simulink model "Drive_Machine"  (R2025a)
settings: Solver=ode23s  StartTime=0.0  StopTime=0.5  MaxStep=1e-5  RelTol=1e-3  AbsTol=1e-3  EnableMultiTasking=on
values from neighbouring files (symbols this model uses):
  f_r = 20    [ISCAD_Analytical.m]
  mparams = load_json_parameters('../ISCAD_parameters.json')    [ISCAD_Analytical.m]    (also in ISCAD_Coupled_Model.m = struct(); PowerElectronics_Analytical.m = load_json_parameters('../TEST_parameters.json'); load_json_parameters.m = struct(); simulik_parameter_setter_inverter.m = load_json_parameters('../TEST_parameters.json'))
  Td = 2e-6    (= 2e-06)    [PowerElectronics_Analytical.m]    (also in simulik_parameter_setter_inverter.m)
  Vs_rms = 0.03    [ISCAD_Analytical.m]
undefined symbols (not defined in the file or in its folder): inv, mach, mi_idx, omega_idx, T, T_sample
libraries: nesl_utility x14, fl_lib x11, ee_lib x5, eePwmGeneratorTwoLevel x1, spsRMSLib x1, simulink x1, spsThreePhaseSineGeneratorLib x1
Description:
  | Three-Phase Voltage-Sourced Converter (SPWM)
  | 
  | This example shows how to model a three-phase voltage-sourced
  | converter that uses Sinusoidal Pulse-Width Modulation (SPWM).
  | This modulation scheme compares a reference sine wave with a
  | higher-frequency repeating triangle wave in order to generate the
  | pulses. The model can be used to support selection of suitable
  | values for L, C and the pulse modulation scheme parameters.
settings Model: Creator=The MathWorks, Inc.  LastModifiedBy=aj22365
settings SolverCC: AutoScaleAbsTol=off  ZeroCrossAlgorithm=Adaptive  AlgebraicLoopSolver=TrustRegion
settings DataIOCC: LimitDataPoints=on  SaveFormat=Array  ReturnWorkspaceOutputs=off
settings OptimizationCC: LifeSpan=inf
settings DebuggingCC: UnderspecifiedInitializationDetection=Classic  MergeDetectMultiDrivingBlocksExec=none  IgnoredZcDiagnostic=none  SolverPrmCheckMsg=warning  UnconnectedInputMsg=warning  UnconnectedOutputMsg=warning  UnconnectedLineMsg=warning  PregeneratedLibrarySubsystemCodeDiagnostic=none  SFUnexpectedBacktrackingDiag=warning  SFNoUnconditionalDefaultTransitionDiag=warning  SFExecutionAtInitializationDiag=none  ArithmeticOperatorsInVariantConditions=warning
settings HardwareCC: ProdBitPerPointer=32.0  ProdBitPerSizeT=32.0  ProdBitPerPtrDiffT=32.0  ProdLargestAtomicFloat=None  ProdIntDivRoundTo=Undefined  ProdEndianess=Unspecified  ProdWordSize=32.0  ProdHWDeviceType=32-bit Generic
settings ModelReferenceCC: EnableRefExpFcnMdlSchedulingChecks=on  PropagateSignalLabelsOutOfModel=off
settings SFSimCC: SimUseLocalCustomCode=off  CustomCodeUndefinedFunction=UseInterfaceOnly
settings RTWCC: RTWUseLocalCustomCode=off  GPUComputeCapability=3.5
settings CodeAppCC: StateflowObjectComments=on
settings GRTTargetCC: TargetLangStandard=C89/C90 (ANSI)
settings ConfigComp: CovMetricSettings=dw  CovSaveCumulativeToWorkspaceVar=on  CovSaveSingleToWorkspaceVar=on  CovExternalEMLEnable=off  CovSFcnEnable=off
settings SimscapeCC: SimscapeNormalizeSystem=off

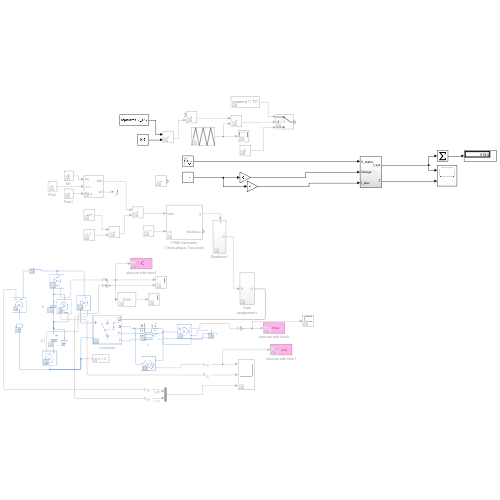
[thumbnail: Simulink's stored preview of the top-level diagram]
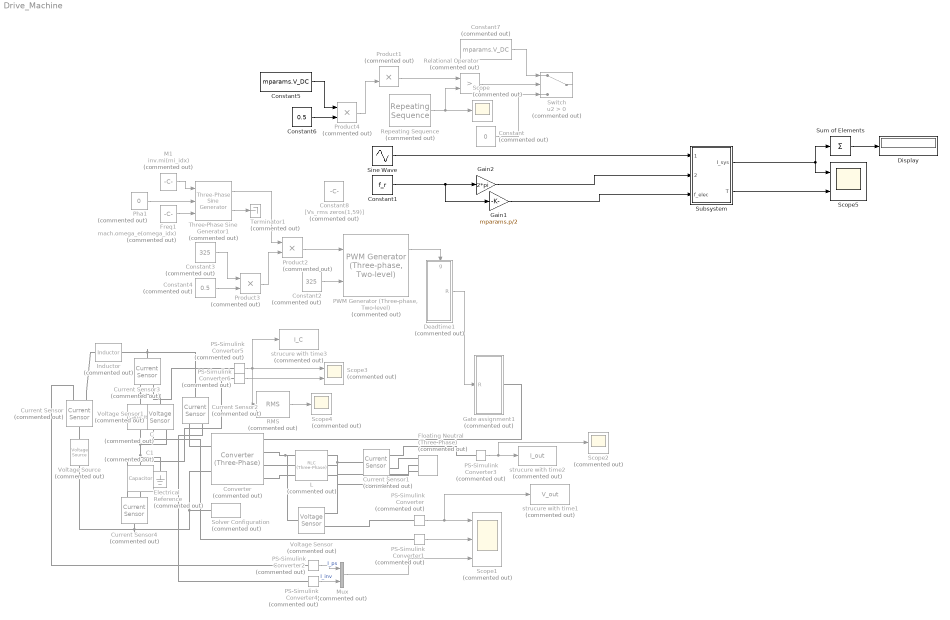
== system Drive_Machine ==
  C : fl_lib/Electrical/Electrical Elements/Capacitor  Commented=on  c=5000 uF  r=0 Ohm  g=0 1/Ohm  i_specify=off  i_priority=High  i=0 A  i_nominal_specify=off  i_nominal_value=1  i_nominal_unit=A  v_specify=on  v_priority=None  v=46 V  v_nominal_specify=off  v_nominal_value=1  v_nominal_unit=V  vc_specify=off  vc_priority=High  vc=0 V  vc_nominal_specify=off  vc_nominal_value=1  vc_nominal_unit=V
  C1 : fl_lib/Electrical/Electrical Elements/Capacitor  Commented=on  c=5000 uF  r=0 Ohm  g=0 1/Ohm  i_specify=off  i_priority=High  i=0 A  i_nominal_specify=off  i_nominal_value=1  i_nominal_unit=A  v_specify=on  v_priority=None  v=46 V  v_nominal_specify=off  v_nominal_value=1  v_nominal_unit=V  vc_specify=off  vc_priority=High  vc=0 V  vc_nominal_specify=off  vc_nominal_value=1  vc_nominal_unit=V
  Constant : Constant  Commented=on  Value=0
  Constant1 : Constant  Value=f_r
  Constant2 : Constant  Commented=on  Value=325
  Constant3 : Constant  Commented=on  Value=325
  Constant4 : Constant  Commented=on  Value=0.5
  Constant5 : Constant  Value=mparams.V_DC
  Constant6 : Constant  Value=0.5
  Constant7 : Constant  Commented=on  Value=mparams.V_DC
  Constant8 : Constant  Commented=on  Value=[Vs_rms zeros(1,59)]
  Converter : ee_lib/Semiconductors & Converters/Converters/Converter (Three-Phase)  Commented=on  port_option=ee.enum.threePhasePort.expanded  fidelity_option=ee.enum.converters.fidelity.detailed  device_type=ee.enum.converters.switchingdevice.igbt  showThermalPort=false  K=0  Vth=0.5 V  Vgt=0.5 V  Vgt_off=0.1 V  Ih=1 A  Vf=0.6 V  Ron=0.002 Ohm  Rds=0.002 Ohm  Goff=1e-6 S  Eon_scalar=22.86e-3 J  Eoff_scalar=17.14e-3 J  Eoff_natural_commutation=10e-3 J  Voff=300 V  Iout_scalar=600 A  onCurrentMeasDelay=0 s  useCurrentFromPreviousCycle=false  useVoltageFromPreviousCycle=false  diode_param=2  diode_Vf=0.8 V  diode_Ron=0.001 Ohm  diode_Goff=1e-5 S  diode_C=5e-8 F  diode_iRM=-235 A  diode_iF=300 A  diode_idot=-50 A/us  diode_trr_param=1  diode_trr_factor=3  diode_trr=15 us  diode_Qrr=1.5e+3 s*uA  diode_rec_loss_model=ee.enum.diode.reverseRecoveryModel.fixed  diode_ErecVal=0 J  diode_scaleWithIandV=false  diode_ErecMat=zeros(2, 3) J  diode_TjrecVec=[298.15, 398.15] K  diode_IfrecVec=[.1, 1, 10] A  diode_IrecVal=10 A  diode_VrecVal=10 V  diode_tFilter=1 / 1000 / 100 s  thermal_network_parameterization=ee.enum.thermalNetworkTopology.external  Rth=[.08, .5] K/W  Rth_Cauer=[.08, .1, .5] K/W  Rth_Foster=[.08, .14, .22, .16] K/W  thermal_mass_parameterization=ee.enum.thermalNetwork.timeconstant  thermal_mass=[.01, .5] J/K  thermal_mass_Cauer=[.01, .1, .5] J/K  thermal_mass_Foster=[.001, .005, .05, .5] J/K  thermal_time_constant=[.001, .2] s  thermal_time_constant_Cauer=[.001, .1, .2] s  thermal_time_constant_Foster=[7e-05, .0007, .01, .08] s  thermal_mass_initial_temperatures=[25, 25] degC  thermal_mass_initial_temperatures_Cauer=[25, 25, 25] degC  junction_thermal_mass=0.01 J/K  Tvec_initial_Foster=[25, 25, 25, 25] degC  snubber_type=0  Cs=1e-7 F  Rs=0.1 Ohm  Vce_loss=[0, 150, 300] V
      settings: InternalSimscapePortConfiguration="{\"Bottom\":[],\"Left\":[{\"id\":\"G\",\"label\":\"G\",\"type\":\"foundation.electrical.twelve_phase\"},{\"id\":\"a\",\"label\":\"a\",\"type\":\"foundation.electrical.electrical\"},{\"id\":\"b\",\"label\":\"b\",\"type\":\"foundation.electrical.electrical\"},{\"id\":\"c\",\"label\":\"c\",\"type\":\"foundation.electrical.electrical\"}],\"Right\":[{\"id\":\"p\",\"label\":\"+\",\"type\":\"foundation.electrical.electrical\"},{\"id\":\"n\",\"label\":\"-\",\"type\":\"foundation.electrical.electrical\"}],\"Top\":[]}"
  Current Sensor{,1..4} (5 alike) : fl_lib/Electrical/Electrical Sensors/Current Sensor  Commented=on
  Deadtime1 : Subsystem  Commented=on
      settings: PortSchema="{\"entries\":[{\"content\":{\"sides\":[{\"content\":{\"connectorIds\":[\"Out1\"]},\"type\":\"ConnectorPlacement.EquallySpacedRectSide\",\"uuid\":\"80ef36b9-f465-4fcc-93a9-9d6eab044ae8\"},{\"content\":{\"side\":\"RIGHT\"},\"type\":\"ConnectorPlacement.EquallySpacedRectSide\",\"uuid\":\"10827d79-0026-467d-af8f-e653363972a6\"},{\"content\":{\"connectorIds\":[\"In1\"],\"side\":\"TOP\"},\"type\":\"ConnectorPlacement.EquallySpacedRectSide\",\"uuid\":\"d9163dac-283f-4784-a2ff-48ce53974a1a\"}]},\"type\":\"ConnectorPlacement.EquallySpacedConnector\",\"uuid\":\"7e643ad6-bdf3-49e0-97a6-0ece4f3a3f1f\"}],\"packageUris\":[\"http://schema.mathworks.com/mf0/Connector/R2020b\"],\"version\":\"1.0\"}"
  Display : Display
  Electrical Reference : fl_lib/Electrical/Electrical Elements/Electrical Reference  Commented=on
  Floating Neutral (Three-Phase) : ee_lib/Connectors & References/Floating Neutral (Three-Phase)  Commented=on  G_parasitic=1e-12 1/Ohm
      settings: InternalSimscapePortConfiguration="{\"Bottom\":[],\"Left\":[{\"id\":\"a\",\"label\":\"a\",\"type\":\"foundation.electrical.electrical\"},{\"id\":\"b\",\"label\":\"b\",\"type\":\"foundation.electrical.electrical\"},{\"id\":\"c\",\"label\":\"c\",\"type\":\"foundation.electrical.electrical\"}],\"Right\":[],\"Top\":[]}"
  Freq1 : Constant  Commented=on  Value=mach.omega_e(omega_idx)
  Gain1 : Gain  Gain=mparams.p/2
  Gain2 : Gain  Gain=2*pi
  Gate assignment1 : Subsystem  Commented=on
  Inductor : fl_lib/Electrical/Electrical Elements/Inductor  Commented=on  l=0.000008 H  r=0.05 Ohm  g=1e-9 1/Ohm  i_specify=on  i_priority=None  i=2 A  i_nominal_specify=off  i_nominal_value=1  i_nominal_unit=A  v_specify=off  v_priority=None  v=0 V  v_nominal_specify=off  v_nominal_value=1  v_nominal_unit=V  i_L_specify=on  i_L_priority=High  i_L=2 A  i_L_nominal_specify=off  i_L_nominal_value=1  i_L_nominal_unit=A
  L : ee_lib/Passive/RLC Assemblies/RLC (Three-Phase)  Commented=on  port_option=ee.enum.threePhasePort.expanded  component_structure=4  R=.054 Ohm  L=.00285 H  C=1e-6 F  R_parasitic=1e-6 Ohm  G_parasitic=1e-6 1/Ohm  IL_specify=on  IL_priority=High  IL=[ -14 7 7 ] A  IL_nominal_specify=off  IL_nominal_value=1  IL_nominal_unit=A  VC_specify=on  VC_priority=High  VC=[ 0 0 0 ] V  VC_nominal_specify=off  VC_nominal_value=1  VC_nominal_unit=V
      settings: InternalSimscapePortConfiguration="{\"Bottom\":[],\"Left\":[{\"id\":\"a1\",\"label\":\"a1\",\"type\":\"foundation.electrical.electrical\"},{\"id\":\"b1\",\"label\":\"b1\",\"type\":\"foundation.electrical.electrical\"},{\"id\":\"c1\",\"label\":\"c1\",\"type\":\"foundation.electrical.electrical\"}],\"Right\":[{\"id\":\"a2\",\"label\":\"a2\",\"type\":\"foundation.electrical.electrical\"},{\"id\":\"b2\",\"label\":\"b2\",\"type\":\"foundation.electrical.electrical\"},{\"id\":\"c2\",\"label\":\"c2\",\"type\":\"foundation.electrical.electrical\"}],\"Top\":[]}"
  M1 : Constant  Commented=on  Value=inv.mi(mi_idx)
  Mux : Mux  Commented=on  Inputs=2
  PS-Simulink Converter{,1..6} (7 alike) : nesl_utility/PS-Simulink Converter  Commented=on  PhysicalDomain=network_engine_domain  SubClassName=ps_output  LeftPortType=input  RightPortType=output  PseudoPeriodic=off  Frequencies=[]  VectorFormat=inherit  Unit=inherit  AffineConversion=off
  "PWM Generator (Three-phase, Two-level)" : eePwmGeneratorTwoLevel/PWM Generator (Three-phase, Two-level)  Commented=on  PWMMode=Continuous PWM (CPWM)  CPWMMode=SPWM: sinusoidal PWM  DPWMMode=30 DPWM: 30 degree discontinuous PWM  fsw=f_s  Ts=T
      settings: SamplingMode=Asymmetric
      settings: LibrarySourceBlock=|
      | ee_sl_lib/Pulse Width
      | Modulation/PWM Generator
      | (Three-phase, Two-level)
  Pha1 : Constant  Commented=on  Value=0
  Product{1..4} (4 alike) : Product  Commented=on
  RMS : spsRMSLib/RMS  Commented=on  TrueRMS=on  Freq=25  RMSInit=0  Ts=inv.T_s
  Relational Operator : RelationalOperator  Commented=on  Operator=>  OutDataTypeStr=boolean  RndMeth=Simplest  InputSameDT=off
  Repeating Sequence : simulink/Sources/Repeating Sequence  Commented=on  rep_seq_t=[0, 1/mparams.f_sw/2, 1/mparams.f_sw]  rep_seq_y=[-1, 1, -1]
  Scope : Scope  Commented=on
      settings: ActiveDisplayYMinimum=-1.25  ActiveDisplayYMaximum=1.25  DataLoggingVariableName=ScopeData3
  Scope1 : Scope  Commented=on  NumInputPorts=3
      settings: ActiveDisplayYMinimum=-286.10507  ActiveDisplayYMaximum=270.03945
  Scope2 : Scope  Commented=on
      settings: ActiveDisplayYMinimum=-372.34194  ActiveDisplayYMaximum=490.06934  DataLoggingVariableName=ScopeData2
  Scope3 : Scope  Commented=on  NumInputPorts=2
      settings: ActiveDisplayYMinimum=-411.29295  ActiveDisplayYMaximum=631.29859
  Scope4 : Scope  Commented=on
      settings: ActiveDisplayYMinimum=-372.34194  ActiveDisplayYMaximum=490.06934
  Scope5 : Scope  NumInputPorts=2
      settings: ActiveDisplayYMinimum=-2.2013460421337228  ActiveDisplayYMaximum=19.812114379203507
  Sine Wave : Sin  Amplitude=Vs_rms*sqrt(2)/mparams.V_DC  Bias=2*Vs_rms*sqrt(2)/mparams.V_DC  Frequency=f_r*mparams.p/2  Phase=[(0:(mparams.Qs-1))*2*pi/60]'  SampleTime=0  VectorParams1D=off
  Solver Configuration : nesl_utility/Solver Configuration  Commented=on  PhysicalDomain=network_engine_domain  SubClassName=solver  LeftPortType=input  RightPortType=generic  Tones=[]  Harmonics=[]  SimulateNoise=off  Profile=off  UseLocalSampling=off  EnableSwitchedLinearOptims=on  FrequencyDomain=off  UseCCode=off  RelTol=0.001  AbsTol=1e-06  MinStep=1e-09  ToWorkspace=off  RevertToSquareIcSolve=off  NumHomotopyIterations=100  PhasorMode=off  PhasorModeNumHarmonics=1  ConsistencySolver=NEWTON_FTOL  IndexReductionMethod=DerivativeReplacement  DoDC=off  ResidualTolerance=1e-09  ConsistencyTolSource=GLOBAL  ConsistencyAbsTol=0.001  ConsistencyRelTol=0.001  ConsistencyTolFactor=0.001  UseLocalSolver=off  LocalSolverChoice=NE_BACKWARD_EULER_ADVANCER  ResolveIndetEquations=on  FunctionEvalNumThread=1  LocalSolverSampleTime=1e-5  DoFixedCost=off  MaxNonlinIter=5  MaxModeIter=2  ComputeImpulses=off  ImpulseIterations=2  LinearAlgebra=Sparse  LinearAlgebraNumThread=0  EquationFormulation=NE_TIME_EF  DelaysMemoryBudget=1024  AutomaticFiltering=on  FilteringTimeConstant=0.001  PartitionStorageMethod=AS_NEEDED  PartitionMemoryBudget=1024  PartitionMethod=FAST  MultibodyUseLocalSolver=off  MultibodyLocalSolverChoice=ODE1  MultibodyLocalSolverSampleTime=0.001
  Subsystem : Subsystem
  Sum of Elements : Sum  Inputs=+
  Switch : Switch  Commented=on  Criteria=u2 > Threshold  SaturateOnIntegerOverflow=off  InputSameDT=off
  Terminator1 : Terminator  Commented=on
  Three-Phase Sine Generator1 : spsThreePhaseSineGeneratorLib/Three-Phase Sine Generator  Commented=on  Ts=T
      settings: LibrarySourceBlock=|
      | sps_lib/Sources/Signal Generator Sources/Three-Phase
      | Sine Generator
  Voltage Sensor : fl_lib/Electrical/Electrical Sensors/Voltage Sensor  Commented=on
  Voltage Sensor1 : fl_lib/Electrical/Electrical Sensors/Voltage Sensor  Commented=on
  Voltage Source : ee_lib/Sources/Voltage Source  Commented=on  dc_voltage=325 V  ac_voltage=0 V  ac_shift=0 rad  ac_frequency=0 Hz  noise_mode=ee.enum.sources.noise.Disabled  PSD=0 V^2/Hz  sample_time=1e-3 s  repeatability=ee.enum.sources.repeatability.NotRepeatable  user_seed=0  auto_seed=3890346746  i_specify=off  i_priority=None  i=0 A  i_nominal_specify=off  i_nominal_value=1  i_nominal_unit=A  v_specify=off  v_priority=None  v=0 V  v_nominal_specify=off  v_nominal_value=1  v_nominal_unit=V
  strucure with time1 : ToWorkspace  Commented=on  VariableName=V_out  SaveFormat=Structure With Time  SampleTime=T_sample
  strucure with time2 : ToWorkspace  Commented=on  VariableName=I_out  SaveFormat=Structure With Time  SampleTime=T_sample
  strucure with time3 : ToWorkspace  Commented=on  VariableName=I_C  SaveFormat=Structure With Time  SampleTime=T_sample
  wires:
  Pha1/1 -> Three-Phase Sine Generator1/2
  Constant2/1 -> "PWM Generator (Three-phase, Two-level)"/2
  Product3/1 -> Product2/2
  Freq1/1 -> Three-Phase Sine Generator1/3
  Constant4/1 -> Product3/2
  Three-Phase Sine Generator1/2 -> Terminator1/1
  M1/1 -> Three-Phase Sine Generator1/1
  Product2/1 -> "PWM Generator (Three-phase, Two-level)"/1
  Constant3/1 -> Product3/1
  Three-Phase Sine Generator1/1 -> Product2/1
  PS-Simulink Converter/1 -> strucure with time1/1, Scope1/1
  Deadtime1/1(R) -> Gate assignment1/1(R)
  "PWM Generator (Three-phase, Two-level)"/1 -> Deadtime1/1(g)
  PS-Simulink Converter1/1 -> Scope1/2
  PS-Simulink Converter3/1 -> Scope2/1, strucure with time2/1
  PS-Simulink Converter4/1 -> Mux/2  "I_inv"
  PS-Simulink Converter2/1 -> Mux/1  "I_ps"
  Mux/1 -> Scope1/3
  PS-Simulink Converter6/1 -> Scope3/2
  PS-Simulink Converter5/1 -> strucure with time3/1, RMS/1, Scope3/1
  RMS/1 -> Scope4/1
  Constant1/1 -> Gain1/1, Gain2/1
  Sum of Elements/1 -> Display/1
  Subsystem/1(I_sys) -> Sum of Elements/1, Scope5/1
  Gain2/1 -> Subsystem/2(Omega)
  Gain1/1 -> Subsystem/3(f_elec)
  Subsystem/2(T) -> Scope5/2
  Constant6/1 -> Product4/2
  Constant5/1 -> Product4/1
  Product4/1 -> Product1/2
  Product1/1 -> Relational Operator/1
  Repeating Sequence/1 -> Scope/1, Relational Operator/2
  Constant7/1 -> Switch/1
  Constant/1 -> Switch/3
  Relational Operator/1 -> Switch/2
  Sine Wave/1 -> Subsystem/1(V_stator)
  connections:
  Converter/LConn2 -- Voltage Sensor/LConn1 -- L/LConn1
  Voltage Sensor/RConn2 -- L/RConn1 -- Current Sensor1/LConn1
  Converter/LConn3 -- L/LConn2
  Converter/LConn4 -- L/LConn3
  Floating Neutral (Three-Phase)/LConn2 -- L/RConn2
  Floating Neutral (Three-Phase)/LConn3 -- L/RConn3
  Gate assignment1/RConn1 -- Converter/LConn1
  Solver Configuration/RConn1 -- Current Sensor4/LConn1 -- Voltage Source/RConn1 -- Converter/RConn2
  C/RConn1 -- Voltage Sensor1/RConn2 -- Electrical Reference/LConn1 -- C1/LConn1
  Voltage Sensor/RConn1 -- PS-Simulink Converter/LConn1
  Current Sensor2/LConn1 -- Inductor/RConn1 -- Current Sensor3/LConn1
  PS-Simulink Converter1/LConn1 -- Voltage Sensor1/RConn1
  Current Sensor/LConn1 -- Voltage Source/LConn1
  Current Sensor/RConn2 -- Inductor/LConn1
  Current Sensor/RConn1 -- PS-Simulink Converter2/LConn1
  Floating Neutral (Three-Phase)/LConn1 -- Current Sensor1/RConn2
  PS-Simulink Converter3/LConn1 -- Current Sensor1/RConn1
  Current Sensor2/RConn2 -- Converter/RConn1
  Current Sensor2/RConn1 -- PS-Simulink Converter4/LConn1
  Voltage Sensor1/LConn1 -- Current Sensor3/RConn2 -- C/LConn1
  Current Sensor4/RConn2 -- C1/RConn1
  PS-Simulink Converter5/LConn1 -- Current Sensor3/RConn1
  Current Sensor4/RConn1 -- PS-Simulink Converter6/LConn1

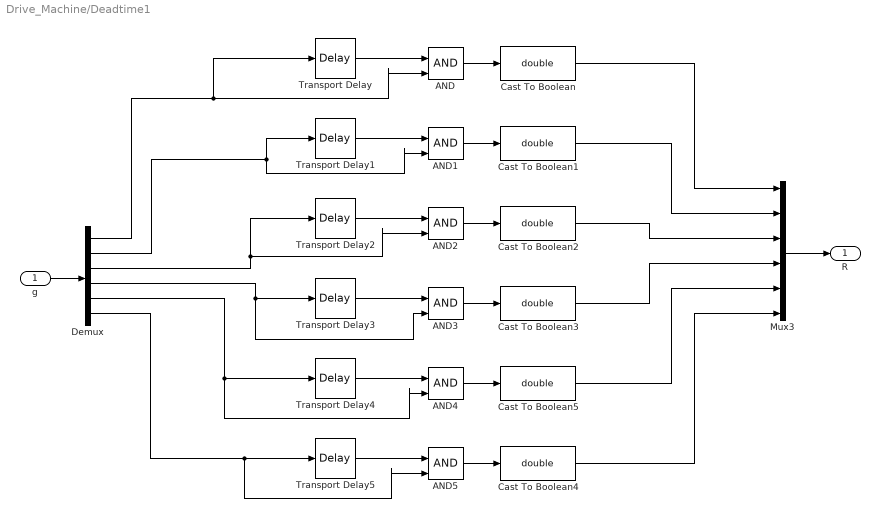
== system Drive_Machine/Deadtime1 ==
  g : Inport
  AND{,1..5} (6 alike) : Logic  IconShape=distinctive  AllPortsSameDT=off  OutDataTypeStr=boolean
  Cast To Boolean{,1..5} (6 alike) : DataTypeConversion  OutDataTypeStr=double  SaturateOnIntegerOverflow=off  RndMeth=Floor
  Demux : Demux  Outputs=6
  Mux3 : Mux  Inputs=6
  Transport Delay{,1..5} (6 alike) : TransportDelay  DelayTime=Td
  R : Outport
  wires:
  g/1 -> Demux/1
  Transport Delay/1 -> AND/1
  Demux/1 -> Transport Delay/1, AND/2
  AND/1 -> Cast To Boolean/1
  Demux/2 -> Transport Delay1/1, AND1/2
  Transport Delay1/1 -> AND1/1
  Transport Delay2/1 -> AND2/1
  AND2/1 -> Cast To Boolean2/1
  Demux/3 -> Transport Delay2/1, AND2/2
  Demux/4 -> AND3/2, Transport Delay3/1
  Transport Delay3/1 -> AND3/1
  Demux/5 -> AND4/2, Transport Delay4/1
  Transport Delay4/1 -> AND4/1
  AND4/1 -> Cast To Boolean5/1
  Demux/6 -> AND5/2, Transport Delay5/1
  Transport Delay5/1 -> AND5/1
  AND1/1 -> Cast To Boolean1/1
  AND3/1 -> Cast To Boolean3/1
  AND5/1 -> Cast To Boolean4/1
  Cast To Boolean/1 -> Mux3/1
  Cast To Boolean1/1 -> Mux3/2
  Cast To Boolean2/1 -> Mux3/3
  Cast To Boolean3/1 -> Mux3/4
  Cast To Boolean5/1 -> Mux3/5
  Cast To Boolean4/1 -> Mux3/6
  Mux3/1 -> R/1

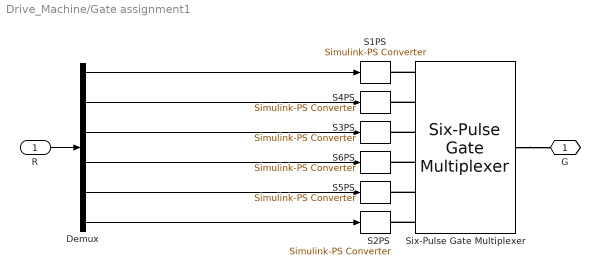
== system Drive_Machine/Gate assignment1 ==
  R : Inport
  Demux : Demux  Outputs=6
  S1PS : nesl_utility/Simulink-PS Converter  PhysicalDomain=network_engine_domain  SubClassName=ps_input  LeftPortType=input  RightPortType=output  PseudoPeriodic=off  Frequencies=[]  NoiseDistribution=none  NoiseParameters=[]  Unit=1  AffineConversion=off  FilteringAndDerivatives=zero  SimscapeFilterOrder=1  InputFilterTimeConstant=.001  UdotUserProvided=1
  S2PS : nesl_utility/Simulink-PS Converter  PhysicalDomain=network_engine_domain  SubClassName=ps_input  LeftPortType=input  RightPortType=output  PseudoPeriodic=off  Frequencies=[]  NoiseDistribution=none  NoiseParameters=[]  Unit=1  AffineConversion=off  FilteringAndDerivatives=zero  SimscapeFilterOrder=1  InputFilterTimeConstant=.001  UdotUserProvided=[]
  S3PS : nesl_utility/Simulink-PS Converter  PhysicalDomain=network_engine_domain  SubClassName=ps_input  LeftPortType=input  RightPortType=output  PseudoPeriodic=off  Frequencies=[]  NoiseDistribution=none  NoiseParameters=[]  Unit=1  AffineConversion=off  FilteringAndDerivatives=zero  SimscapeFilterOrder=1  InputFilterTimeConstant=.001  UdotUserProvided=[]
  S4PS : nesl_utility/Simulink-PS Converter  PhysicalDomain=network_engine_domain  SubClassName=ps_input  LeftPortType=input  RightPortType=output  PseudoPeriodic=off  Frequencies=[]  NoiseDistribution=none  NoiseParameters=[]  Unit=1  AffineConversion=off  FilteringAndDerivatives=zero  SimscapeFilterOrder=1  InputFilterTimeConstant=.001  UdotUserProvided=[]
  S5PS : nesl_utility/Simulink-PS Converter  PhysicalDomain=network_engine_domain  SubClassName=ps_input  LeftPortType=input  RightPortType=output  PseudoPeriodic=off  Frequencies=[]  NoiseDistribution=none  NoiseParameters=[]  Unit=1  AffineConversion=off  FilteringAndDerivatives=zero  SimscapeFilterOrder=1  InputFilterTimeConstant=.001  UdotUserProvided=[]
  S6PS : nesl_utility/Simulink-PS Converter  PhysicalDomain=network_engine_domain  SubClassName=ps_input  LeftPortType=input  RightPortType=output  PseudoPeriodic=off  Frequencies=[]  NoiseDistribution=none  NoiseParameters=[]  Unit=1  AffineConversion=off  FilteringAndDerivatives=zero  SimscapeFilterOrder=1  InputFilterTimeConstant=.001  UdotUserProvided=[]
  Six-Pulse Gate Multiplexer : ee_lib/Semiconductors & Converters/Converters/Six-Pulse Gate Multiplexer  port_option=ee.enum.controlport.ps
  G : PMIOPort  Side=Right
  wires:
  R/1 -> Demux/1
  Demux/1 -> S1PS/1
  Demux/2 -> S4PS/1
  Demux/3 -> S3PS/1
  Demux/4 -> S6PS/1
  Demux/5 -> S5PS/1
  Demux/6 -> S2PS/1
  connections:
  Six-Pulse Gate Multiplexer/LConn1 -- S1PS/RConn1
  Six-Pulse Gate Multiplexer/LConn2 -- S4PS/RConn1
  Six-Pulse Gate Multiplexer/RConn1 -- G/RConn1
  Six-Pulse Gate Multiplexer/LConn3 -- S3PS/RConn1
  Six-Pulse Gate Multiplexer/LConn6 -- S2PS/RConn1
  Six-Pulse Gate Multiplexer/LConn5 -- S5PS/RConn1
  Six-Pulse Gate Multiplexer/LConn4 -- S6PS/RConn1

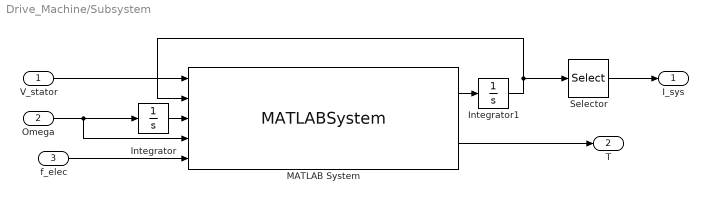
== system Drive_Machine/Subsystem ==
  V_stator : Inport
  Omega : Inport  Port=2
  f_elec : Inport  Port=3
  Integrator : Integrator
  Integrator1 : Integrator  InitialCondition=zeros(mparams.Qs+mparams.Qr,1)
  MATLAB System : MATLABSystem  System=ISCAD_Coupled_Model  mparams=struct()  Resolution_Factor=10  f_sw=mparams.f_sw  Qs=mparams.Qs  Qr=mparams.Qr  p=mparams.p  rho_s=mparams.rho_s  h_slot=mparams.h_slot  ag=mparams.ag  l_stack=mparams.l_stack  w_slot=mparams.w_slot  r=mparams.r  h_so=mparams.h_so  w_so=mparams.w_so  Ts=1e-6  SimulateUsing=Code generation
      mask Type: ISCAD_Coupled_Model
  Selector : Selector  InputPortWidth=mparams.Qs+mparams.Qr  IndexOptions=Index vector (dialog)  Indices=[1:mparams.Qs]  OutputSizes=1
  I_sys : Outport
  T : Outport  Port=2
  wires:
  f_elec/1 -> MATLAB System/5
  Integrator1/1 -> Selector/1, MATLAB System/2
  MATLAB System/1 -> Integrator1/1
  Omega/1 -> Integrator/1, MATLAB System/4
  V_stator/1 -> MATLAB System/1
  MATLAB System/2 -> T/1
  Integrator/1 -> MATLAB System/3
  Selector/1 -> I_sys/1
